simulink subsystem "rocket_plant"  (R2024b)
settings: Solver=VariableStepAuto  StartTime=0.0  StopTime=10.0  RelTol=1e-3
values from neighbouring files (symbols this model uses):
  Mdot = [-2.06885767428 -2.65545019236 -3.15692906995 -3.53463604631 -3.77514336449 -3.88832803946 -3.9029455228 -3.85572128709 -3.78250824721 -3.71051505737 -3.65407665098 -3.61686646614 ... (1300 elements, 1300x1)]    [barrowaman.mat]
  rail_angle = 0.0872664625997    [barrowaman.mat]
  sim_time = [0.01 0.02 0.03 0.04 0.05 0.06 0.07 0.08 0.09 0.1 0.11 0.12 ... (1300 elements, 1300x1)]    [barrowaman.mat]
libraries: shared6dof x1
settings Model: Creator=joedo  LastModifiedBy=trist

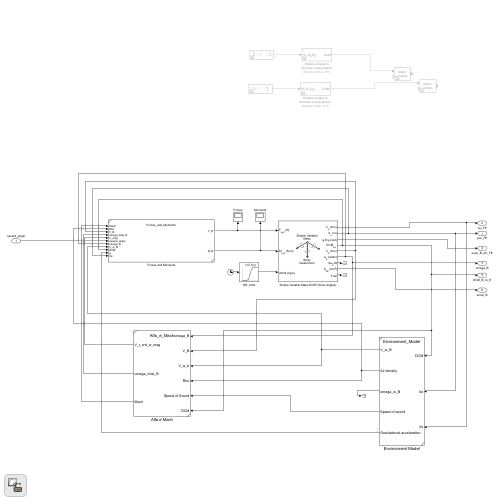
[thumbnail: Simulink's stored preview of the top-level diagram]
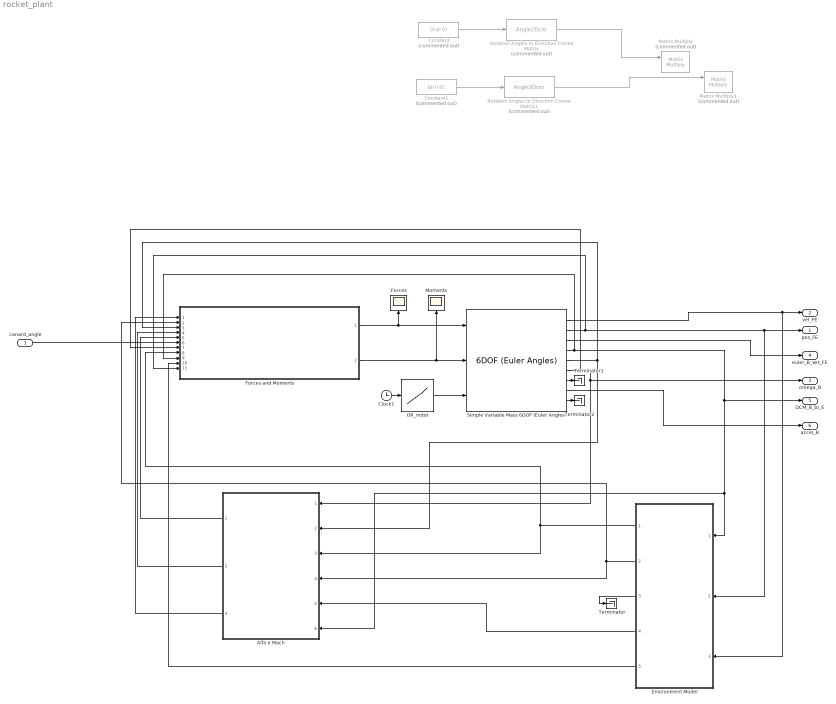
== system rocket_plant ==
  canard_angle : Inport
  Alfa e Mach : Subsystem  ReferencedSubsystem=Alfa_e_Mach
  Clock1 : Clock
  Constant : Constant  Commented=on  Value=[0 pi 0]
  Constant1 : Constant  Commented=on  Value=[pi 0 0]
  Environment Model : Subsystem  ReferencedSubsystem=Environment_Model
  Forces : Scope
  "Forces and Moments " : Subsystem  ReferencedSubsystem=Forces_and_Moments
  Matrix Multiply : Product  Commented=on  Multiplication=Matrix(*)
  Matrix Multiply1 : Product  Commented=on  Multiplication=Matrix(*)
  Moments : Scope
  OR_mdot : Lookup_n-D  NumberOfTableDimensions=1  BreakpointsForDimension1=sim_time  Table=Mdot  InternalRulePriority=Speed  RndMeth=Simplest
  Rotation Angles to Direction Cosine Matrix : Angle2Dcm  Commented=on
      settings: AttributesFormatString=Rotation Order: %<rotationOrder>
  Rotation Angles to Direction Cosine Matrix1 : Angle2Dcm  Commented=on
      settings: AttributesFormatString=Rotation Order: %<rotationOrder>
  Simple Variable Mass 6DOF (Euler Angles) : shared6dof/6DOF (Euler Angles)  units=Metric (MKS)  mtype=Simple Variable  rep=Quaternion  xme_0=[0 0 0]  Vm_0=[0 0 0]  eul_0=[0 -pi/2+rail_angle 0]  pm_0=[0 0 0]  mass_0=total_mass_0  mass_e=total_mass_d  mass_f=total_mass_0  inertia=eye(3)  inertia_e=I_d  inertia_f=I_0  k_quat=1.0  vre_flag=off  abi_flag=off  aMode=aMode  xme_statename=''  Vm_statename=''  eul_statename=''  quat_statename=''  pm_statename=''  mass_statename=''
  Terminator : Terminator
  Terminator1 : Terminator
  Terminator2 : Terminator
  pos_FE : Outport
  vel_FE : Outport  Port=2
  omega_B : Outport  Port=3
  euler_B_wrt_FE : Outport  Port=4
  DCM_B_to_E : Outport  Port=5
  accel_B : Outport  Port=6
  wires:
  "Forces and Moments "/1 -> Forces/1, Simple Variable Mass 6DOF (Euler Angles)/1
  Alfa e Mach/1 -> "Forces and Moments "/5
  canard_angle/1 -> "Forces and Moments "/6
  Simple Variable Mass 6DOF (Euler Angles)/4 -> Alfa e Mach/6, Environment Model/1, DCM_B_to_E/1, "Forces and Moments "/9
  Simple Variable Mass 6DOF (Euler Angles)/6 -> Alfa e Mach/1, omega_B/1, "Forces and Moments "/7
  Simple Variable Mass 6DOF (Euler Angles)/5 -> Alfa e Mach/2, "Forces and Moments "/3
  Environment Model/1 -> Alfa e Mach/3, "Forces and Moments "/8
  Alfa e Mach/2 -> "Forces and Moments "/4
  Environment Model/2 -> Alfa e Mach/4, "Forces and Moments "/2
  "Forces and Moments "/2 -> Moments/1, Simple Variable Mass 6DOF (Euler Angles)/2
  Environment Model/4 -> Alfa e Mach/5
  Simple Variable Mass 6DOF (Euler Angles)/2 -> "Forces and Moments "/11, Environment Model/2, pos_FE/1
  Alfa e Mach/3 -> "Forces and Moments "/1
  Simple Variable Mass 6DOF (Euler Angles)/7 -> Terminator1/1
  OR_mdot/1 -> Simple Variable Mass 6DOF (Euler Angles)/3
  Simple Variable Mass 6DOF (Euler Angles)/8 -> accel_B/1
  Simple Variable Mass 6DOF (Euler Angles)/9 -> Terminator2/1
  Environment Model/5 -> "Forces and Moments "/10
  Constant1/1 -> Rotation Angles to Direction Cosine Matrix1/1
  Constant/1 -> Rotation Angles to Direction Cosine Matrix/1
  Rotation Angles to Direction Cosine Matrix1/1 -> Matrix Multiply1/1
  Rotation Angles to Direction Cosine Matrix/1 -> Matrix Multiply/1
  Clock1/1 -> OR_mdot/1
  Simple Variable Mass 6DOF (Euler Angles)/1 -> Environment Model/3, vel_FE/1
  Simple Variable Mass 6DOF (Euler Angles)/3 -> euler_B_wrt_FE/1
  Environment Model/3 -> Terminator/1
